simulink model "DCMotorStateFlow"  (R2020b)
settings: Solver=VariableStepAuto  StartTime=0.0  StopTime=10.0  RelTol=1e-3
settings Model: Creator=yuto  LastModifiedBy=yuto

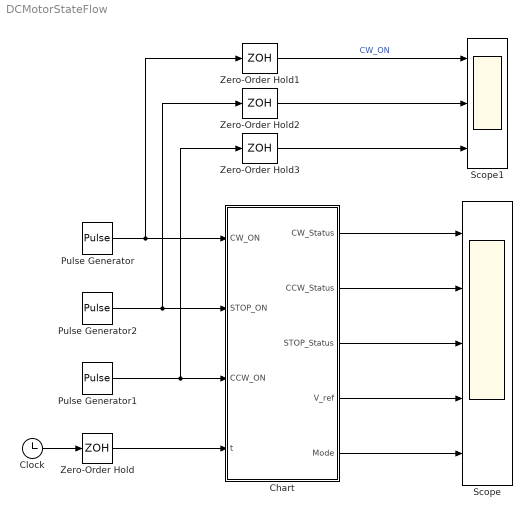
== system DCMotorStateFlow ==
  Chart : Stateflow chart  TreatAsAtomicUnit=on
  Clock : Clock
  Pulse Generator : DiscretePulseGenerator  PulseType=Time based  Period=10  PulseWidth=5
  Pulse Generator1 : DiscretePulseGenerator  PulseType=Time based  Period=10  PulseWidth=5
  Pulse Generator2 : DiscretePulseGenerator  PulseType=Time based  Period=10  PulseWidth=5
  Scope : Scope  NumInputPorts=5
  Scope1 : Scope  NumInputPorts=3
  Zero-Order Hold{,1..3} (4 alike) : ZeroOrderHold  SampleTime=-1
  wires:
  Pulse Generator/1 -> Zero-Order Hold1/1, Chart/1(CW_ON)
  Pulse Generator2/1 -> Zero-Order Hold2/1, Chart/2(STOP_ON)
  Pulse Generator1/1 -> Zero-Order Hold3/1, Chart/3(CCW_ON)
  Clock/1 -> Zero-Order Hold/1
  Zero-Order Hold/1 -> Chart/4(t)
  Chart/1(CW_Status) -> Scope/1
  Chart/2(CCW_Status) -> Scope/2
  Chart/3(STOP_Status) -> Scope/3
  Chart/4(V_ref) -> Scope/4
  Chart/5(Mode) -> Scope/5
  Zero-Order Hold1/1 -> Scope1/1  "CW_ON"
  Zero-Order Hold2/1 -> Scope1/2
  Zero-Order Hold3/1 -> Scope1/3

== stateflow chart DCMotorStateFlow/Chart ==
  state CW
    state Accel
    state Stedy
    state DeAccel
    (default) -> CW.Accel
    CW.Accel -> CW.Stedy
    CW.Stedy -> CW.Accel [order 1]
    CW.Stedy -> CW.DeAccel [order 2]
    CW.DeAccel -> CW.Stedy
  state STOP
    entry:
    Mode=0;
    y = 0;
    STOP = 1;
    during:
    y=0;
    exit:
    STOP=0;
  state CCW
    state Accel
    state Stedy
    state DeAccel
    (default) -> CCW.Accel
    CCW.Accel -> CCW.Stedy
    CCW.Stedy -> CCW.Accel [order 1]
    CCW.Stedy -> CCW.DeAccel [order 2]
    CCW.DeAccel -> CCW.Stedy
  (default) -> STOP
  CW -> STOP : [Co1]
  STOP -> CW [order 1] : [Co2]
  CCW -> STOP : [Co4]
  STOP -> CCW [order 2] : [Co3]
  data: CW_ON input; STOP_ON input; CCW_ON input; t input; CW_Status output; CCW_Status output; STOP_Status output; V_ref output; Mode output
